simulink model "questao24"  (R2020b)
settings: Solver=VariableStepAuto  StartTime=0.0  StopTime=15  RelTol=1e-3
settings Model: Creator=lucas  LastModifiedBy=lucas

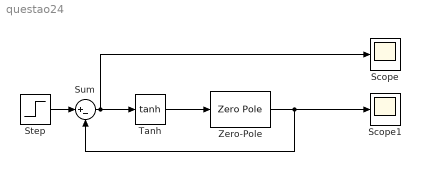
== system questao24 ==
  Scope : Scope
  Scope1 : Scope
  Step : Step  SampleTime=0
  Sum : Sum  Inputs=|+-
  Tanh : Trigonometry  Operator=tanh
  Zero-Pole : ZeroPole  Zeros=[]  Poles=[0 -1]
  wires:
  Tanh/1 -> Zero-Pole/1
  Step/1 -> Sum/1
  Sum/1 -> Scope/1, Tanh/1
  Zero-Pole/1 -> Scope1/1, Sum/2
